simulink library "canblocks_extras"  (Simulink 7.6)
settings: Solver=ode45  SolverMode=SingleTasking  StartTime=0.0  StopTime=10.0  RelTol=1e-3
undefined symbols (not defined in the file or in its folder): CCP_STATION_ID, TOTAL_NUM_ODTS
libraries: canblocks_extras x1, config_library x1
settings Model: Creator=The MathWorks Inc.

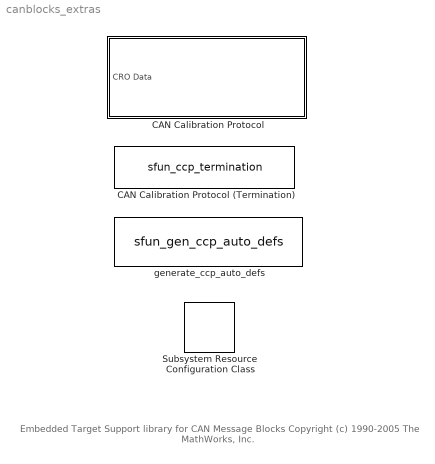
== system canblocks_extras ==
  note: Embedded Target
      | Support library for CAN Message Blocks
      | Copyright (c) 1990-2005 The MathWorks, Inc.
  CAN Calibration Protocol : Subsystem  mask(CAN Calibration Protocol (Target-side)){CCP_STATION_ID=CCP_STATION_ID, TOTAL_NUM_ODTS=TOTAL_NUM_ODTS, show_commands=off, GET_CCP_VERSIONenabled=on, EXCHANGE_IDenabled=on, SET_MTAenabled=on, DNLOADenabled=on, DNLOAD_6enabled=on, UPLOADenabled=on, SHORT_UPenabled=on, GET_DAQ_SIZEenabled=on, SET_DAQ_PTRenabled=on, WRITE_DAQenabled=on, START_STOPenabled=on, SET_S_STATUSenabled=on, GET_S_STATUSenabled=on, START_STOP_ALLenabled=on}
      mask prompts: CCP_STATION_ID "CAN station address (16-bit integer):"; TOTAL_NUM_ODTS "Total Number of ODTs"; show_commands "Enable / Disable Connected State Commands"; GET_CCP_VERSIONenabled "GET_CCP_VERSION"; EXCHANGE_IDenabled "EXCHANGE_ID"; SET_MTAenabled "SET_MTA"; DNLOADenabled "DNLOAD"; DNLOAD_6enabled "DNLOAD_6"; UPLOADenabled "UPLOAD"; SHORT_UPenabled "SHORT_UP"; GET_DAQ_SIZEenabled "GET_DAQ_SIZE"; SET_DAQ_PTRenabled "SET_DAQ_PTR"; WRITE_DAQenabled "WRITE_DAQ"; START_STOPenabled "START_STOP"; SET_S_STATUSenabled "SET_S_STATUS"; GET_S_STATUSenabled "GET_S_STATUS"; START_STOP_ALLenabled "START_STOP_ALL"
      mask help:
      | Implements a subset of the CAN Calibration Protocol (CCP v2.1) on the target processor.
      |
      | This block processes a Command Receive Object (CRO) and outputs the resulting Data Transmission Object (DTO).
      mask init:
      | % resource config - make sure
      | % only a single CCP block is in each
      | % target subsystem
      | mask_resource_validator(gcb,@canblocks_ccp_validate, 'CCP_BLOCK');
      settings: AttributesFormatString=\n\n
      mask Help: helpview([docroot '/toolbox/can_blocks/can_blocks.map'], 'target_CCP');
      mask CallbackString: ||ccp_init_mask('show_commands_mask_callback',gcb);||||||||||||||
      mask Display:
      | disp('CCP Kernel');
      | 
      | port_label('input',1, 'CRO Data');
  CAN Calibration Protocol (Termination) : S-Function  FunctionName=sfun_ccp_termination  EnableBusSupport=off
      mask Display: disp('CCP Termination');
  Subsystem Resource Configuration Class : config_library/Subsystem Resource Configuration Class  Tag=CONFIGURATION DATA CLASS  SystemSampleTime=-1  dClassName=TargetsCommonConfig.CCP  rClassName=TargetsCommonConfig.CCP_RESOURCES
  generate_ccp_auto_defs : S-Function  FunctionName=sfun_gen_ccp_auto_defs  EnableBusSupport=off
      mask Display: disp('Append comment to ccp_auto_defs.h');

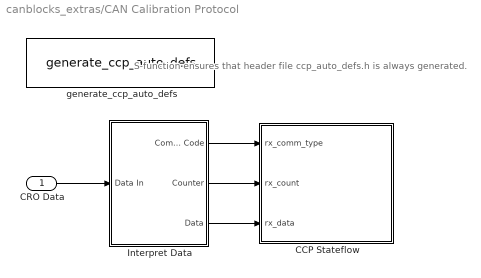
== system canblocks_extras/CAN Calibration Protocol ==
  note: S-function ensures that
      | header file ccp_auto_defs.h
      | is always generated.
  CRO Data : Inport
  "CCP Stateflow " : Stateflow chart  TreatAsAtomicUnit=on
  Interpret Data : Subsystem
  generate_ccp_auto_defs : canblocks_extras/generate_ccp_auto_defs
  wires:
  Interpret Data/1(Command Code) -> "CCP Stateflow "/1(rx_comm_type)
  Interpret Data/2(Counter) -> "CCP Stateflow "/2(rx_count)
  Interpret Data/3(Data) -> "CCP Stateflow "/3(rx_data)
  CRO Data/1 -> Interpret Data/1(Data In)

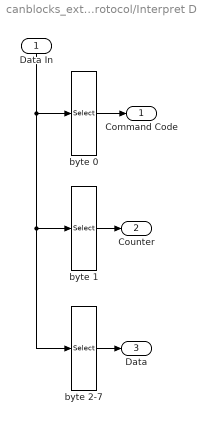
== system canblocks_extras/CAN Calibration Protocol/Interpret Data ==
  Data In : Inport
  byte 0 : Selector  InputPortWidth=8  IndexOptions=Index vector (dialog)  Indices=1  OutputSizes=1
  byte 1 : Selector  InputPortWidth=8  IndexOptions=Index vector (dialog)  Indices=2  OutputSizes=1
  byte 2-7 : Selector  InputPortWidth=8  IndexOptions=Index vector (dialog)  Indices=3:8  OutputSizes=1
  Command Code : Outport
  Counter : Outport  Port=2
  Data : Outport  Port=3
  wires:
  byte 0/1 -> Command Code/1
  byte 1/1 -> Counter/1
  byte 2-7/1 -> Data/1
  Data In/1 -> byte 2-7/1, byte 1/1, byte 0/1

== stateflow chart CAN Calibration Protocol/CCP Stateflow  ==
  settings: sampleTime=1  executeAtInitialization=1
  state tx_dto(tx_comm_type) [function]
    note: Flag to other blocks that this block could deal with the command.
    note: Returns the Slave CCP Version.
    note: No Slave ID implementation +
        | Mem. Programming and DAQ available (No Cal) +
        | all are unlocked.
    note: Returns the current mta -
        | using get_mta()
    note: Returns data read from the target. From specified address.
    note: Returns data read from the target. Using MTA.
    note: // S_STATUS_QUALIFIER is 0
        | we do not use additional status info.
        | The session status info is returned in byte 4.
    (default) -> (junction 51) : {setHandled(1);
        | setData(0,CCP_DTO_ID);
        | setData(1,CCP_CRC_OK);
        | setData(2,command_counter);
        | }
    (junction 51) -> (junction 52) [order 1] : [tx_comm_type==CCP_TEST]
    (junction 52) -> (junction 53)
    (junction 51) -> (junction 55) [order 2]
    (junction 53) -> (junction 54) : {setData(3,0);setData(4,0);setData(5,0);
        | setData(6,0);setData(7,0);}
    (junction 56) -> (junction 53)
    (junction 58) -> (junction 53)
    (junction 60) -> (junction 53)
    (junction 62) -> (junction 53)
    (junction 64) -> (junction 53)
    (junction 66) -> (junction 53)
    (junction 68) -> (junction 53)
    (junction 70) -> (junction 53)
    (junction 55) -> (junction 56) [order 1] : [tx_comm_type==CCP_DISCONNECT]
    (junction 55) -> (junction 57) [order 2]
    (junction 57) -> (junction 58) [order 1] : [tx_comm_type==CCP_CONNECT]
    (junction 57) -> (junction 59) [order 2]
    (junction 59) -> (junction 60) [order 1] : [tx_comm_type==CCP_SET_MTA]
    (junction 59) -> (junction 61) [order 2]
    (junction 61) -> (junction 62) [order 1] : [tx_comm_type==CCP_SET_DAQ_PTR]
    (junction 61) -> (junction 63) [order 2]
    (junction 63) -> (junction 64) [order 1] : [tx_comm_type==CCP_WRITE_DAQ]
    (junction 63) -> (junction 65) [order 2]
    (junction 65) -> (junction 66) [order 1] : [tx_comm_type==CCP_START_STOP]
    (junction 65) -> (junction 67) [order 2]
    (junction 67) -> (junction 68) [order 1] : [tx_comm_type==CCP_START_STOP_ALL]
    (junction 67) -> (junction 69) [order 2]
    (junction 69) -> (junction 70) [order 1] : [tx_comm_type==CCP_SET_S_STATUS]
    (junction 69) -> (junction 71) [order 2]
    (junction 71) -> (junction 72) [order 1] : [tx_comm_type==CCP_GET_CCP_VERSION]
        | {setData(3,getSlave_Version(0));
        | setData(4,getSlave_Version(1));}
    (junction 71) -> (junction 73) [order 2]
    (junction 73) -> (junction 74) [order 1] : [tx_comm_type==CCP_EXCHANGE_ID]
        | {setData(3,SLAVE_ID_LENGTH_NOT_USED);
        | setData(4,SLAVE_ID_DATA_TYPE_NOT_USED);
        | setData(5,RESOURCE_AVAILABILITY_MASK);
        | setData(6,RESOURCE_PROTECTION_MASK);}
    (junction 73) -> (junction 75) [order 2]
    (junction 75) -> (junction 76) [order 1] : [(tx_comm_type==CCP_DNLOAD) || (tx_comm_type==CCP_DNLOAD_6)]
        | {setData(3,MTA_ADDRESS_EXTENSION);
        | get_mta0(4);}
    (junction 75) -> (junction 77) [order 2]
    (junction 77) -> (junction 78) [order 1] : [tx_comm_type==CCP_SHORT_UPLOAD]
        | {c_setUINT32bytes(&memptr, &rx_data[2]);
        | c_read_uint8s(getDataPtr(3),rx_data[0], &memptr);}
    (junction 77) -> (junction 79) [order 2]
    (junction 79) -> (junction 80) [order 1] : [tx_comm_type==CCP_UPLOAD]
        | {c_read_uint8s(getDataPtr(3),rx_data[0],getMTAPtr(0));}
    (junction 79) -> (junction 81) [order 2]
    (junction 81) -> (junction 82) [order 1] : [tx_comm_type==CCP_GET_DAQ_SIZE]
        | {c_init_daq_list(rx_data[0]);
        | setData(5,0);setData(6,0);setData(7,0);
        | }
    (junction 81) -> (junction 83) [order 2]
    (junction 83) -> (junction 84) : [tx_comm_type==CCP_GET_S_STATUS]
        | { setData(3,getS_Status());
        |  setData(4,S_STATUS_QUALIFIER);}
  state get_mta0(first_byte) [function]
    note: Copy the MTA (byte by byte) into the output array, dout.
        | Note: This is Endian independent.   The Endianess achieved
        | is that of the processor executing the kernel.
    (default) -> (junction 85) : {c_getUINT32bytes(getMTAPtr(0), getDataPtr(first_byte));}
  state write_daq() [function]
    (default) -> (junction 86) : {c_setUINT32bytes(&address, &rx_data[2]);
        | c_write_daq(rx_data[0],address);}
  state set_mta() [function]
    note: Copy the input array, rx_data (byte by byte) into the appropriate MTA.
        | Note: This is Endian independent.  The Endianess achieved is that
        | of the processor executing the kernel.
    note: NOTE: rx_data[0] == MTA Number - either 0 or 1.
    (default) -> (junction 87) : {c_setUINT32bytes(getMTAPtr(rx_data[0]),&rx_data[2]);}
  state init() [function]
    note: Initialisation of the kernel
    (default) -> (junction 89) : {setSlave_Version(0,2);
        | setSlave_Version(1,1);
        | setStation_Address(0,uint8(CCP_STATION_ID & 0xFF));
        | setStation_Address(1,uint8(CCP_STATION_ID >> 8));}
  state unhandled_command() [function]
    (default) -> (junction 90) : {setHandled(0);
        | setData(0,rx_comm_type);
        | setData(1, rx_count);
        | setData(2 , rx_data[0]);
        | setData(3, rx_data[1]);
        | setData(4, rx_data[2]);
        | setData(5, rx_data[3]);
        | setData(6, rx_data[4]);
        | setData(7, rx_data[5]);}
  state Disconnected/
    entry:setCurrent_State(CCP_DISCONNECTED_STATE);
    entry:c_reset_all_DAQ_lists();
    note: 2 possible commands when disconnected.  Each command has the station
        | address as an argument.   Local var. 'station address' is stored in Intel(LE) format.
    note: Acknowledge the test.
    note: Master must be communicating with a different
        | Slave.
    note: Not in connected state so any blocks further down the chain will not do anything.
    note: Go into connected state.
    note: NOTE: On entry to this state, all DAQ lists are reset and
        | data transmission stops.
        | This is PERMANENT DISCONNECT.
        |
        | NOTE: SET_SESSION_STATUS "resume bit" is NOT
        | supported and DAQ related functions are reset.
    Disconnected -> (junction 92) : {command_counter=rx_count;}
    (junction 92) -> (junction 91) [order 3] : {setHandled(0);}
    (junction 92) -> (junction 93) [order 2] : [rx_comm_type==CCP_TEST &&...
        | rx_data[0]==getStation_Address(0) &&...
        | rx_data[1]==getStation_Address(1)]
        | {tx_dto(CCP_TEST);}
  state Temporarily_Disconnected/
    entry:setCurrent_State(CCP_TEMPORARILY_DISCONNECTED_STATE);
    note: Check station address for test.
    note: Valid connect.
    note: Master must be communicating with a different Slave.
    note: Not in connected state so any blocks further down the chain will not do anything.
    note: NOTE: On entry into this state,
        | all DAQ lists are maintained
        | and data transmission continues.
        | This is TEMPORARY DISCONNECT.
    Temporarily_Disconnected -> (junction 94) : {command_counter=rx_count;}
    (junction 94) -> (junction 95)
    (junction 95) -> (junction 96) [order 1] : [rx_comm_type==CCP_TEST&&...
        | rx_data[0]==getStation_Address(0)&&...
        | rx_data[1]==getStation_Address(1)]...
        | {tx_dto(CCP_TEST);}
    (junction 95) -> (junction 97) [order 2]
    (junction 97) -> (junction 98) [order 2] : {setHandled(0);}
  state Connected/
    entry:setCurrent_State(CCP_CONNECTED_STATE);
    note: Exit CONNECTED STATE
        | Permanent Disconnect
    note: Exit CONNECTED STATE
        | Temporary Disconnect
    note: When DAQ lists are implemented, perhaps they
        | should be reset here.
    note: For this implementation, we just record
        | the info. given by the master.
    note: Call set_mta to initialize the appropriate MTA pointer.
    note: Write up to 5 bytes to memory.
    note: Read up to 5 bytes from memory.
    note: Must be an unrecognised command.
        | Set the command as unhandled so
        | blocks further down the chain can
        | handle it.
    note: Clear a DAQ list and find it's size.
    note: Init. the DAQ list pointer.
    note: Writes one entry (element) to a DAQ list.
    note: store the session status
    note: return the session status
    note: Acknowledge TEST to this Station Address
    note: Acknowledge CONNECT to this Station Address
    note: Leaving connected state
        | so any blocks further down
        | the chain will not do anything.
    note: Leaving connected state
        | so any blocks further down
        | the chain will not do anything.
    Connected -> (junction 99) : {command_counter=rx_count;}
    (junction 99) -> (junction 100) [order 1] : [GET_CCP_VERSIONenabled && (rx_comm_type==CCP_GET_CCP_VERSION)]
        | {setMaster_Version(0,rx_data[0]);
        | setMaster_Version(1,rx_data[1]);
        | tx_dto(CCP_GET_CCP_VERSION);}
    (junction 99) -> (junction 101) [order 2]
    (junction 101) -> (junction 102) [order 1] : [EXCHANGE_IDenabled && (rx_comm_type==CCP_EXCHANGE_ID)]
        | {tx_dto(CCP_EXCHANGE_ID);}
    (junction 101) -> (junction 103) [order 2]
    (junction 103) -> (junction 104) [order 1] : [SET_MTAenabled && (rx_comm_type==CCP_SET_MTA)]
        | {set_mta();
        | tx_dto(CCP_SET_MTA);}
    (junction 103) -> (junction 105) [order 2]
    (junction 105) -> (junction 106) [order 1] : [DNLOADenabled && (rx_comm_type==CCP_DNLOAD)]
        | {c_write_uint8s(&rx_data[1], rx_data[0], getMTAPtr(0));
        | tx_dto(CCP_DNLOAD);}
    (junction 105) -> (junction 107) [order 2]
    (junction 107) -> (junction 108) [order 1] : [DNLOAD_6enabled && (rx_comm_type==CCP_DNLOAD_6)]
        | {c_write_uint8s(&rx_data[0],6,getMTAPtr(0));
        | tx_dto(CCP_DNLOAD_6);}
    (junction 107) -> (junction 109) [order 2]
    (junction 109) -> (junction 110) [order 1] : [SHORT_UPenabled && (rx_comm_type==CCP_SHORT_UPLOAD)]
        | {tx_dto(CCP_SHORT_UPLOAD);}
    (junction 109) -> (junction 111) [order 2]
    (junction 111) -> (junction 112) [order 1] : [UPLOADenabled && (rx_comm_type==CCP_UPLOAD)]
        | {tx_dto(CCP_UPLOAD);}
    (junction 111) -> (junction 113) [order 2]
    (junction 113) -> (junction 114) [order 1] : [GET_DAQ_SIZEenabled && (rx_comm_type==CCP_GET_DAQ_SIZE)]
        | {tx_dto(CCP_GET_DAQ_SIZE);}
    (junction 113) -> (junction 115) [order 2]
    (junction 115) -> (junction 116) [order 1] : [SET_DAQ_PTRenabled && (rx_comm_type==CCP_SET_DAQ_PTR)]
        | {c_set_element_pointer(rx_data[0],rx_data[1],rx_data[2]);
        | tx_dto(CCP_SET_DAQ_PTR);}
    (junction 115) -> (junction 117) [order 2]
    (junction 117) -> (junction 118) [order 1] : [WRITE_DAQenabled && (rx_comm_type==CCP_WRITE_DAQ)]
        | {write_daq();
        | tx_dto(CCP_WRITE_DAQ);}
    (junction 117) -> (junction 119) [order 2]
    (junction 119) -> (junction 120) [order 1] : [START_STOP_ALLenabled && (rx_comm_type==CCP_START_STOP_ALL)]
        | {c_start_stop_all(rx_data[0]);
        | tx_dto(CCP_START_STOP_ALL);}
    (junction 119) -> (junction 121) [order 2]
    (junction 121) -> (junction 122) [order 1] : [START_STOPenabled && (rx_comm_type==CCP_START_STOP)]
        | {c_start_stop(rx_data[0],rx_data[1],rx_data[2],rx_data[3],1);
        | tx_dto(CCP_START_STOP);}
    (junction 121) -> (junction 123) [order 2]
    (junction 123) -> (junction 124) [order 1] : [SET_S_STATUSenabled && (rx_comm_type==CCP_SET_S_STATUS)]
        | {setS_Status(rx_data[0]);
        |  tx_dto(CCP_SET_S_STATUS);}
    (junction 123) -> (junction 125) [order 2]
    (junction 125) -> (junction 126) [order 1] : [GET_S_STATUSenabled && (rx_comm_type==CCP_GET_S_STATUS)]
        | {tx_dto(CCP_GET_S_STATUS);}
    (junction 125) -> (junction 127) [order 2]
    (junction 127) -> (junction 128) [order 1] : [rx_comm_type==CCP_TEST]
    (junction 128) -> (junction 129) [order 1] : [rx_data[0]==getStation_Address(0) &&...
        | rx_data[1]==getStation_Address(1)]
        | {tx_dto(CCP_TEST);}
    (junction 127) -> (junction 130) [order 2]
    (junction 128) -> (junction 136) [order 2] : {setHandled(0);}
    (junction 130) -> (junction 131) [order 1] : [rx_comm_type==CCP_CONNECT]
    (junction 131) -> (junction 132) [order 1] : [rx_data[0]==getStation_Address(0) &&...
        | rx_data[1]==getStation_Address(1)]
        | {tx_dto(CCP_CONNECT);}
    (junction 130) -> (junction 133) [order 2]
    (junction 131) -> (junction 135) [order 2] : {setHandled(0);}
    (junction 133) -> (junction 134) [order 1] : [rx_comm_type==CCP_DISCONNECT]
    (junction 134) -> (junction 135) [order 2] : [rx_data[0]==TEMPORARY_DISCONNECT]
        | {tx_dto(CCP_DISCONNECT);}
    (junction 135) -> (junction 136)
    (junction 133) -> (junction 88) [order 2] : {unhandled_command();}
  (default) -> Disconnected : {init();}
  (junction 92) -> Connected [order 1] : [rx_comm_type==CCP_CONNECT &&...
      | rx_data[0]==getStation_Address(0) &&...
      | rx_data[1]==getStation_Address(1)]
      | /tx_dto(CCP_CONNECT);
  (junction 97) -> Connected [order 1] : [rx_comm_type==CCP_CONNECT &&...
      | rx_data[0]==getStation_Address(0) &&...
      | rx_data[1]==getStation_Address(1)]
      | {tx_dto(CCP_CONNECT);}
  (junction 136) -> Temporarily_Disconnected
  (junction 134) -> Disconnected [order 1] : [rx_data[0]==PERMANENT_DISCONNECT]
      | {tx_dto(CCP_DISCONNECT);}
  data: tx_comm_type function_input uint8; SLAVE_ID_LENGTH_NOT_USED constant uint8; SLAVE_ID_DATA_TYPE_NOT_USED constant uint8; RESOURCE_AVAILABILITY_MASK constant uint8 =66; RESOURCE_PROTECTION_MASK constant uint8; MTA_ADDRESS_EXTENSION constant uint8; S_STATUS_QUALIFIER constant uint8; memptr temporary uint32; first_byte function_input uint8; address temporary uint32; rx_comm_type input uint8; rx_count input uint8; rx_data input uint8 size=6; command_counter local uint8; TEMPORARY_DISCONNECT constant uint8; PERMANENT_DISCONNECT constant uint8 =1; GET_CCP_VERSIONenabled parameter boolean; EXCHANGE_IDenabled parameter boolean; SET_MTAenabled parameter boolean; DNLOADenabled parameter boolean; UPLOADenabled parameter boolean; SHORT_UPenabled parameter boolean; GET_DAQ_SIZEenabled parameter boolean; SET_DAQ_PTRenabled parameter boolean; WRITE_DAQenabled parameter boolean; START_STOPenabled parameter boolean; SET_S_STATUSenabled parameter boolean; GET_S_STATUSenabled parameter boolean; START_STOP_ALLenabled parameter boolean; CCP_STATION_ID parameter uint16; DNLOAD_6enabled parameter boolean
